simulink model "PSO_PDD_OLD"  (R2015a)
settings: Solver=ode4  StartTime=0.0  StopTime=16  FixedStep=0.1  RelTol=1e-3
model workspace: external: MAT-File co-effs.mat (data not in the file)
libraries: aerolibutil x7, vrlib x5, simulink x1, simulink_extras x1
settings Model: Creator=Nick  LastModifiedBy=Nick
settings DataIOCC: ReturnWorkspaceOutputs=on

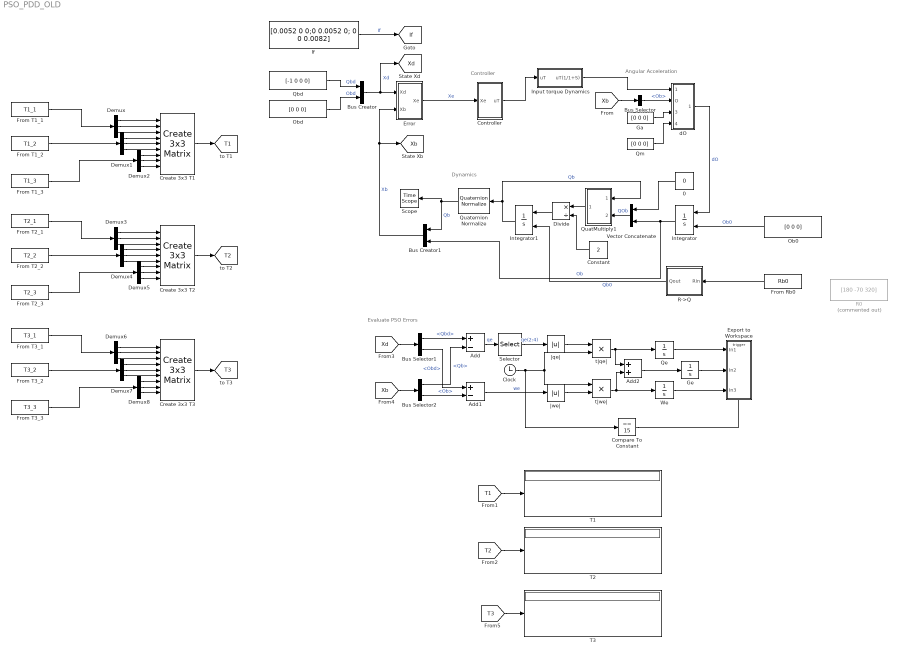
== system PSO_PDD_OLD ==
  note: Evaluate PSO Errors
  note: Dynamics
  note: Controller
  note: Angular Acceleration
  0 : Constant  Value=0
  Add : Sum  Inputs=+-
  Add1 : Sum  Inputs=+-
  Add2 : Sum
  Bus Creator : BusCreator  Inputs='Qbd','Obd'
  Bus Creator1 : BusCreator  Inputs='Qb','Ob'
  Bus Selector : BusSelector  OutputSignals=Ob
  Bus Selector1 : BusSelector  OutputSignals=Qbd,Obd
  Bus Selector2 : BusSelector  OutputSignals=Qb,Ob
  Clock : Clock
  Compare To Constant : simulink/Logic and Bit Operations/Compare To Constant  relop===  const=15  OutDataTypeStr=boolean
  Constant : Constant  Value=2
  Controller : Subsystem
  Create 3x3 T1 : aerolibutil/Create 3x3 Matrix
  Create 3x3 T2 : aerolibutil/Create 3x3 Matrix
  Create 3x3 T3 : aerolibutil/Create 3x3 Matrix
  Demux{,1..8} (9 alike) : Demux  Outputs=3
  Divide : Product  Inputs=*/
  Error : Subsystem
  Export to Workspace : Subsystem
  From Rb0 : FromWorkspace  VariableName=Rb0  SampleTime=0
  From T1_1 : FromWorkspace  VariableName=T1_1  SampleTime=0
  From T1_2 : FromWorkspace  VariableName=T1_2  SampleTime=0
  From T1_3 : FromWorkspace  VariableName=T1_3  SampleTime=0
  From T2_1 : FromWorkspace  VariableName=T2_1  SampleTime=0
  From T2_2 : FromWorkspace  VariableName=T2_2  SampleTime=0
  From T2_3 : FromWorkspace  VariableName=T2_3  SampleTime=0
  From T3_1 : FromWorkspace  VariableName=T3_1  SampleTime=0
  From T3_2 : FromWorkspace  VariableName=T3_2  SampleTime=0
  From T3_3 : FromWorkspace  VariableName=T3_3  SampleTime=0
  Ga : Constant  Value=[0 0 0]
  Ge : Integrator
  If : Constant  Value=[0.0052 0 0;0 0.0052 0; 0 0 0.0082]  VectorParams1D=off
  Input torque Dynamics : Subsystem
  Integrator : Integrator  InitialConditionSource=external
  Integrator1 : Integrator  InitialConditionSource=external
  Ob0 : Constant  Value=[0 0 0]
  Obd : Constant  Value=[0 0 0]
  Qbd : Constant  Value=[-1 0 0 0]
  Qe : Integrator
  Qm : Constant  Value=[0 0 0]
  QuatMultiply1 : Subsystem
  Quaternion Normalize : aerolibutil/Quaternion Normalize
  R->Q : Subsystem
  R0 : Constant  Commented=on  Value=[180 -70 320]
  Scope : TimeScope
  Selector : Selector  InputPortWidth=4  Indices=[2 3 4]
  T1 : Display
  T2 : Display
  T3 : Display
  Vector Concatenate : Concatenate
  We : Integrator
  dO : Subsystem
  t|qe| : Product
  t|we| : Product
  |qe| : Abs
  |we| : Abs
  tag scope: If=global, T1=global, T2=global, T3=global, Xb=global, Xd=global
  wires:
  Qbd/1 -> Bus Creator/1  "Qbd"
  Obd/1 -> Bus Creator/2  "Obd"
  Bus Creator/1 -> [Xd], Error/1(Xd)  "Xd"
  If/1 -> [If]  "If"
  Error/1(Xe) -> Controller/1(Xe)  "Xe"
  Controller/1(uT) -> Input torque Dynamics/1(uT)
  Input torque Dynamics/1(uT(1/1+S)) -> dO/1(uT)
  [Xb] -> Bus Selector/1
  Bus Selector/1 -> dO/2(O)  "<Ob>"
  Ga/1 -> dO/3(Ga)
  Qm/1 -> dO/4(Qm)
  dO/1(dO) -> Integrator/1  "dO"
  Integrator/1 -> Vector Concatenate/2, Bus Creator1/2  "Ob"
  Constant/1 -> Divide/2
  R->Q/1(Qout) -> Integrator1/2  "Qb0"
  Integrator1/1 -> Quaternion Normalize/1, QuatMultiply1/1(Q1 in)  "Qb"
  0/1 -> Vector Concatenate/1
  Vector Concatenate/1 -> QuatMultiply1/2(Q2 in)  "QOb"
  Divide/1 -> Integrator1/1
  QuatMultiply1/1(Qout) -> Divide/1
  Quaternion Normalize/1 -> Bus Creator1/1, Scope/1  "Qb"
  Bus Creator1/1 -> Error/2(Xb), [Xb]  "Xb"
  [Xb] -> Bus Selector2/1
  [Xd] -> Bus Selector1/1
  Bus Selector1/1 -> Add/1  "<Qbd>"
  Bus Selector1/2 -> Add1/1  "<Obd>"
  Bus Selector2/1 -> Add/2  "<Qb>"
  Bus Selector2/2 -> Add1/2  "<Ob>"
  Add/1 -> Selector/1  "qe"
  Clock/1 -> Compare To Constant/1, t|we|/1, t|qe|/2
  t|qe|/1 -> Qe/1, Add2/1
  Selector/1 -> |qe|/1  "qe(2:4)"
  |qe|/1 -> t|qe|/1
  |we|/1 -> t|we|/2
  t|we|/1 -> Add2/2, We/1
  Add1/1 -> |we|/1  "we"
  Add2/1 -> Ge/1
  Qe/1 -> Export to Workspace/1(In1)
  Ge/1 -> Export to Workspace/2(In2)
  We/1 -> Export to Workspace/3(In3)
  Compare To Constant/1 -> Export to Workspace/Trigger
  Ob0/1 -> Integrator/2  "Ob0"
  From Rb0/1 -> R->Q/1(Rin)
  From T1_2/1 -> Demux1/1
  From T1_1/1 -> Demux/1
  From T1_3/1 -> Demux2/1
  Demux/1 -> Create 3x3 T1/1
  Demux/2 -> Create 3x3 T1/2
  Demux/3 -> Create 3x3 T1/3
  Demux1/1 -> Create 3x3 T1/4
  Demux1/2 -> Create 3x3 T1/5
  Demux1/3 -> Create 3x3 T1/6
  Demux2/1 -> Create 3x3 T1/7
  Demux2/2 -> Create 3x3 T1/8
  Demux2/3 -> Create 3x3 T1/9
  Create 3x3 T1/1 -> [T1]
  From T2_2/1 -> Demux4/1
  From T2_1/1 -> Demux3/1
  From T2_3/1 -> Demux5/1
  Demux3/1 -> Create 3x3 T2/1
  Demux3/2 -> Create 3x3 T2/2
  Demux3/3 -> Create 3x3 T2/3
  Demux4/1 -> Create 3x3 T2/4
  Demux4/2 -> Create 3x3 T2/5
  Demux4/3 -> Create 3x3 T2/6
  Demux5/1 -> Create 3x3 T2/7
  Demux5/2 -> Create 3x3 T2/8
  Demux5/3 -> Create 3x3 T2/9
  Create 3x3 T2/1 -> [T2]
  From T3_2/1 -> Demux7/1
  From T3_1/1 -> Demux6/1
  From T3_3/1 -> Demux8/1
  Demux6/1 -> Create 3x3 T3/1
  Demux6/2 -> Create 3x3 T3/2
  Demux6/3 -> Create 3x3 T3/3
  Demux7/1 -> Create 3x3 T3/4
  Demux7/2 -> Create 3x3 T3/5
  Demux7/3 -> Create 3x3 T3/6
  Demux8/1 -> Create 3x3 T3/7
  Demux8/2 -> Create 3x3 T3/8
  Demux8/3 -> Create 3x3 T3/9
  Create 3x3 T3/1 -> [T3]
  [T1] -> T1/1
  [T2] -> T2/1
  [T3] -> T3/1

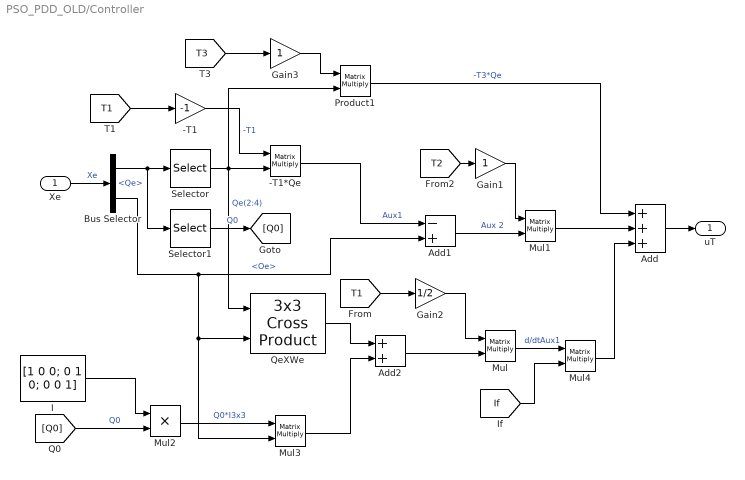
== system PSO_PDD_OLD/Controller ==
  Xe : Inport  PortDimensions=7
  -T1 : Gain  Gain=-1
  -T1*Qe : Product  Multiplication=Matrix(*)
  Add : Sum  Inputs=+++
  Add1 : Sum  Inputs=-+
  Add2 : Sum
  Bus Selector : BusSelector  OutputSignals=Qe,Oe
  Gain1 : Gain
  Gain2 : Gain  Gain=1/2
  Gain3 : Gain
  I : Constant  Value=[1 0 0; 0 1 0; 0 0 1]
  Mul{,1,3..4} (4 alike) : Product  Inputs=**  Multiplication=Matrix(*)
  Mul2 : Product  Inputs=**
  Product1 : Product  Multiplication=Matrix(*)
  QeXWe : aerolibutil/3x3 Cross Product
  Selector : Selector  InputPortWidth=4  Indices=[2 3 4]
  Selector1 : Selector  InputPortWidth=4  Indices=[1]
  uT : Outport  PortDimensions=3
  wires:
  Xe/1 -> Bus Selector/1  "Xe"
  Bus Selector/1 -> Selector1/1, Selector/1  "<Qe>"
  Selector/1 -> Product1/2, -T1*Qe/2, QeXWe/1  "Qe(2:4)"
  [T1] -> -T1/1
  -T1/1 -> -T1*Qe/1  "-T1"
  -T1*Qe/1 -> Add1/1  "Aux1"
  [T2] -> Gain1/1
  Add1/1 -> Mul1/2  "Aux 2"
  Gain1/1 -> Mul1/1
  Mul1/1 -> Add/2
  Bus Selector/2 -> Mul3/2, QeXWe/2, Add1/2  "<Oe>"
  Selector1/1 -> [Q0]  "Q0"
  I/1 -> Mul2/1
  [Q0] -> Mul2/2  "Q0"
  Mul2/1 -> Mul3/1  "Q0*I3x3"
  QeXWe/1 -> Add2/1
  Mul3/1 -> Add2/2
  Add2/1 -> Mul/2
  [T1] -> Gain2/1
  Gain2/1 -> Mul/1
  [T3] -> Gain3/1
  Gain3/1 -> Product1/1
  Product1/1 -> Add/1  "-T3*Qe"
  [If] -> Mul4/2
  Add/1 -> uT/1
  Mul/1 -> Mul4/1  "d/dtAux1"
  Mul4/1 -> Add/3

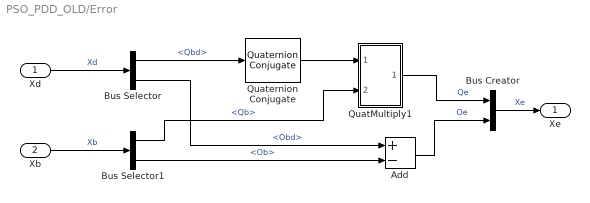
== system PSO_PDD_OLD/Error ==
  Xd : Inport
  Xb : Inport  Port=2  PortDimensions=7
  Add : Sum  Inputs=+-
  Bus Selector : BusSelector  OutputSignals=Qbd,Obd
  Bus Selector1 : BusSelector  OutputSignals=Qb,Ob
  Bus Creator : BusCreator  Inputs=2
  QuatMultiply1 : Subsystem
  Quaternion Conjugate : aerolibutil/Quaternion Conjugate
  Xe : Outport
  wires:
  Xd/1 -> Bus Selector/1  "Xd"
  Xb/1 -> Bus Selector1/1  "Xb"
  Bus Selector/1 -> Quaternion Conjugate/1  "<Qbd>"
  Bus Selector/2 -> Add/1  "<Obd>"
  QuatMultiply1/1(Qout) -> Bus Creator/1  "Qe"
  Add/1 -> Bus Creator/2  "Oe"
  Bus Creator/1 -> Xe/1  "Xe"
  Bus Selector1/1 -> QuatMultiply1/2(Q2 in)  "<Qb>"
  Quaternion Conjugate/1 -> QuatMultiply1/1(Q1 in)
  Bus Selector1/2 -> Add/2  "<Ob>"

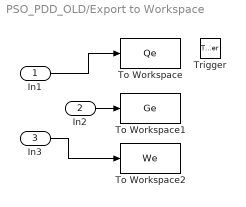
== system PSO_PDD_OLD/Export to Workspace ==
  In1 : Inport
  In2 : Inport  Port=2
  In3 : Inport  Port=3
  Trigger : TriggerPort  PortDimensions=1
  To Workspace : ToWorkspace  VariableName=Qe  SampleTime=-1
  To Workspace1 : ToWorkspace  VariableName=Ge  SampleTime=-1
  To Workspace2 : ToWorkspace  VariableName=We  SampleTime=-1
  wires:
  In1/1 -> To Workspace/1
  In2/1 -> To Workspace1/1
  In3/1 -> To Workspace2/1

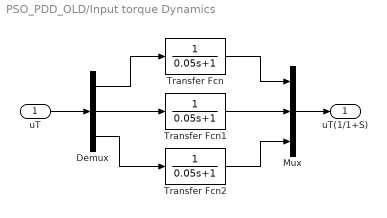
== system PSO_PDD_OLD/Input torque Dynamics ==
  uT : Inport  PortDimensions=3
  Demux : Demux  Outputs=3
  Mux : Mux  Inputs=3
  Transfer Fcn : TransferFcn  Denominator=[0.05 1]
  Transfer Fcn1 : TransferFcn  Denominator=[0.05 1]
  Transfer Fcn2 : TransferFcn  Denominator=[0.05 1]
  uT(1/1+S) : Outport  PortDimensions=3
  wires:
  uT/1 -> Demux/1
  Demux/1 -> Transfer Fcn/1
  Demux/2 -> Transfer Fcn1/1
  Demux/3 -> Transfer Fcn2/1
  Transfer Fcn/1 -> Mux/1
  Transfer Fcn1/1 -> Mux/2
  Transfer Fcn2/1 -> Mux/3
  Mux/1 -> uT(1/1+S)/1

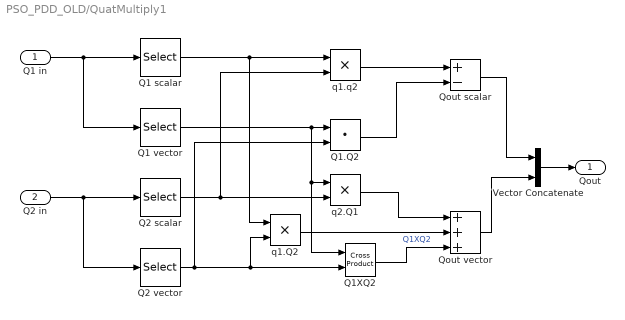
== system PSO_PDD_OLD/QuatMultiply1 ==
  Q1 in : Inport  PortDimensions=[4]
  Q2 in : Inport  Port=2  PortDimensions=[4]
  Q1 scalar : Selector  InputPortWidth=4  Indices=[1]
  Q1 vector : Selector  InputPortWidth=4  Indices=[2 3 4]
  Q1.Q2 : DotProduct  InputSameDT=on  OutDataTypeStr=Inherit: Inherit via internal rule
  Q1XQ2 : vrlib/Utilities/Cross Product
  Q2 scalar : Selector  InputPortWidth=4  Indices=[1]
  Q2 vector : Selector  InputPortWidth=4  Indices=[2 3 4]
  Qout scalar : Sum  Inputs=+-
  Qout vector : Sum  Inputs=+++
  Vector Concatenate : Concatenate
  q1.Q2 : Product
  q1.q2 : Product
  q2.Q1 : Product
  Qout : Outport  PortDimensions=[4]
  wires:
  Q1 in/1 -> Q1 vector/1, Q1 scalar/1
  Q2 in/1 -> Q2 vector/1, Q2 scalar/1
  Q1 scalar/1 -> q1.q2/1, q1.Q2/1
  Q2 scalar/1 -> q1.q2/2, q2.Q1/2
  Q1 vector/1 -> Q1.Q2/1, Q1XQ2/1, q2.Q1/1
  Q2 vector/1 -> Q1.Q2/2, Q1XQ2/2, q1.Q2/2
  q1.q2/1 -> Qout scalar/1
  Q1.Q2/1 -> Qout scalar/2
  q2.Q1/1 -> Qout vector/1
  q1.Q2/1 -> Qout vector/2
  Qout scalar/1 -> Vector Concatenate/1
  Qout vector/1 -> Vector Concatenate/2
  Vector Concatenate/1 -> Qout/1
  Q1XQ2/1 -> Qout vector/3  "Q1XQ2"

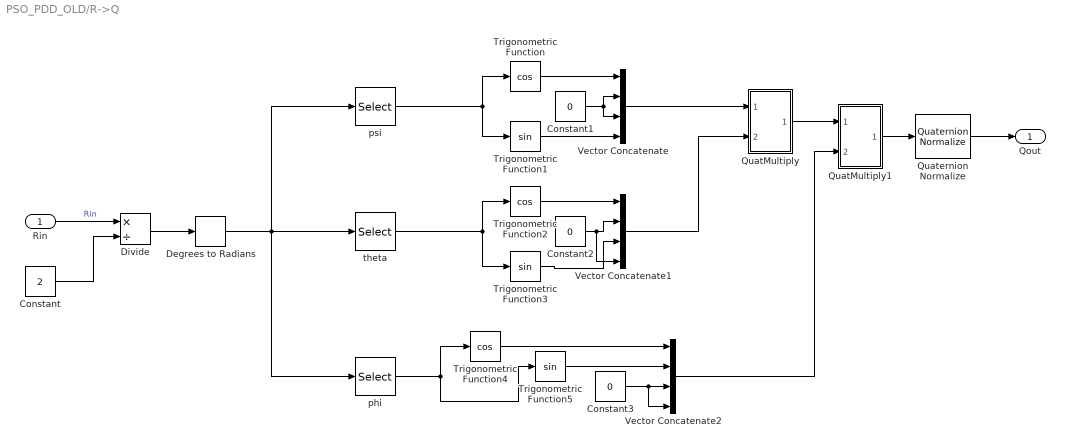
== system PSO_PDD_OLD/R->Q ==
  Rin : Inport  PortDimensions=3
  Constant : Constant  Value=2
  Constant1 : Constant  Value=0
  Constant2 : Constant  Value=0
  Constant3 : Constant  Value=0
  Degrees to Radians : simulink_extras/Transformations/Degrees to Radians
  Divide : Product  Inputs=*/
  QuatMultiply : Subsystem
  QuatMultiply1 : Subsystem
  Quaternion Normalize : aerolibutil/Quaternion Normalize
  Trigonometric Function : Trigonometry  Operator=cos
  Trigonometric Function1 : Trigonometry
  Trigonometric Function2 : Trigonometry  Operator=cos
  Trigonometric Function3 : Trigonometry
  Trigonometric Function4 : Trigonometry  Operator=cos
  Trigonometric Function5 : Trigonometry
  Vector Concatenate : Concatenate  NumInputs=4
  Vector Concatenate1 : Concatenate  NumInputs=4
  Vector Concatenate2 : Concatenate  NumInputs=4
  phi : Selector  InputPortWidth=3  Indices=[1]
  psi : Selector  InputPortWidth=3  Indices=[3]
  theta : Selector  InputPortWidth=3  Indices=[2]
  Qout : Outport  PortDimensions=[4]
  wires:
  Trigonometric Function/1 -> Vector Concatenate/1
  psi/1 -> Trigonometric Function1/1, Trigonometric Function/1
  Trigonometric Function1/1 -> Vector Concatenate/4
  Constant1/1 -> Vector Concatenate/3, Vector Concatenate/2
  Constant/1 -> Divide/2
  Rin/1 -> Divide/1  "Rin"
  Trigonometric Function2/1 -> Vector Concatenate1/1
  theta/1 -> Trigonometric Function3/1, Trigonometric Function2/1
  Constant2/1 -> Vector Concatenate1/4, Vector Concatenate1/2
  Trigonometric Function3/1 -> Vector Concatenate1/3
  Trigonometric Function4/1 -> Vector Concatenate2/1
  phi/1 -> Trigonometric Function5/1, Trigonometric Function4/1
  Trigonometric Function5/1 -> Vector Concatenate2/2
  Constant3/1 -> Vector Concatenate2/4, Vector Concatenate2/3
  Vector Concatenate/1 -> QuatMultiply/1(Q1 in)
  Vector Concatenate1/1 -> QuatMultiply/2(Q2 in)
  QuatMultiply/1(Qout) -> QuatMultiply1/1(Q1 in)
  Vector Concatenate2/1 -> QuatMultiply1/2(Q2 in)
  Divide/1 -> Degrees to Radians/1
  Degrees to Radians/1 -> phi/1, psi/1, theta/1
  QuatMultiply1/1(Qout) -> Quaternion Normalize/1
  Quaternion Normalize/1 -> Qout/1

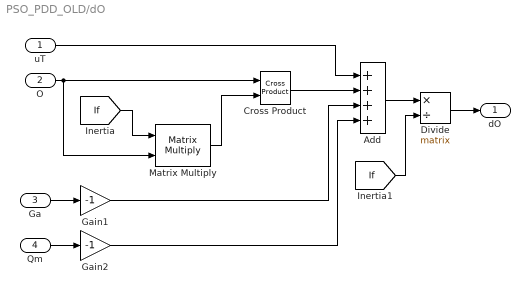
== system PSO_PDD_OLD/dO ==
  uT : Inport  PortDimensions=3
  O : Inport  Port=2  PortDimensions=3
  Ga : Inport  Port=3  PortDimensions=3
  Qm : Inport  Port=4  PortDimensions=3
  Add : Sum  Inputs=++++
  Cross Product : vrlib/Utilities/Cross Product
  Divide : Product  Inputs=*/  Multiplication=Matrix(*)
  Gain1 : Gain  Gain=-1
  Gain2 : Gain  Gain=-1
  Matrix Multiply : Product  Multiplication=Matrix(*)
  dO : Outport  PortDimensions=3
  wires:
  Divide/1 -> dO/1
  [If] -> Divide/2
  Ga/1 -> Gain1/1
  Qm/1 -> Gain2/1
  uT/1 -> Add/1
  Gain1/1 -> Add/3
  Gain2/1 -> Add/4
  Add/1 -> Divide/1
  [If] -> Matrix Multiply/1
  O/1 -> Cross Product/1, Matrix Multiply/2
  Matrix Multiply/1 -> Cross Product/2
  Cross Product/1 -> Add/2

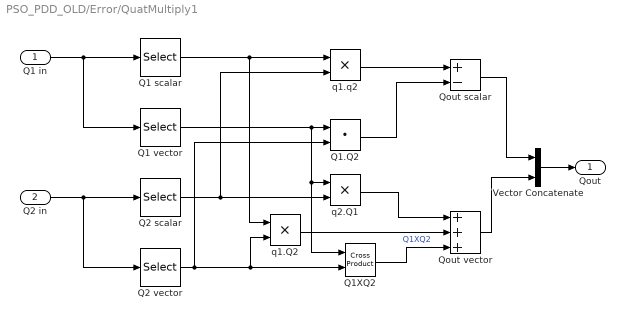
== system PSO_PDD_OLD/Error/QuatMultiply1 ==
  Q1 in : Inport  PortDimensions=[4]
  Q2 in : Inport  Port=2  PortDimensions=[4]
  Q1 scalar : Selector  InputPortWidth=4  Indices=[1]
  Q1 vector : Selector  InputPortWidth=4  Indices=[2 3 4]
  Q1.Q2 : DotProduct  InputSameDT=on  OutDataTypeStr=Inherit: Inherit via internal rule
  Q1XQ2 : vrlib/Utilities/Cross Product
  Q2 scalar : Selector  InputPortWidth=4  Indices=[1]
  Q2 vector : Selector  InputPortWidth=4  Indices=[2 3 4]
  Qout scalar : Sum  Inputs=+-
  Qout vector : Sum  Inputs=+++
  Vector Concatenate : Concatenate
  q1.Q2 : Product
  q1.q2 : Product
  q2.Q1 : Product
  Qout : Outport  PortDimensions=[4]
  wires:
  Q1 in/1 -> Q1 vector/1, Q1 scalar/1
  Q2 in/1 -> Q2 vector/1, Q2 scalar/1
  Q1 scalar/1 -> q1.q2/1, q1.Q2/1
  Q2 scalar/1 -> q1.q2/2, q2.Q1/2
  Q1 vector/1 -> Q1.Q2/1, Q1XQ2/1, q2.Q1/1
  Q2 vector/1 -> Q1.Q2/2, Q1XQ2/2, q1.Q2/2
  q1.q2/1 -> Qout scalar/1
  Q1.Q2/1 -> Qout scalar/2
  q2.Q1/1 -> Qout vector/1
  q1.Q2/1 -> Qout vector/2
  Qout scalar/1 -> Vector Concatenate/1
  Qout vector/1 -> Vector Concatenate/2
  Vector Concatenate/1 -> Qout/1
  Q1XQ2/1 -> Qout vector/3  "Q1XQ2"

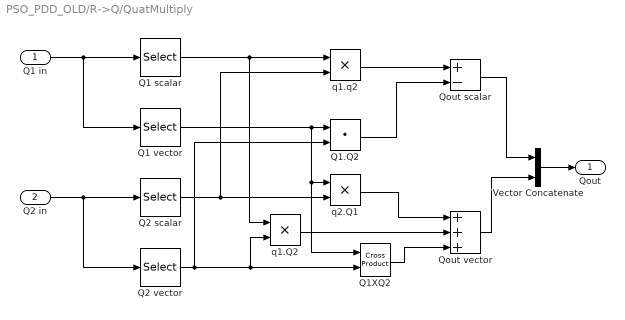
== system PSO_PDD_OLD/R->Q/QuatMultiply ==
  Q1 in : Inport  PortDimensions=[4]
  Q2 in : Inport  Port=2  PortDimensions=[4]
  Q1 scalar : Selector  InputPortWidth=4  Indices=[1]
  Q1 vector : Selector  InputPortWidth=4  Indices=[2 3 4]
  Q1.Q2 : DotProduct  InputSameDT=on  OutDataTypeStr=Inherit: Inherit via internal rule
  Q1XQ2 : vrlib/Utilities/Cross Product
  Q2 scalar : Selector  InputPortWidth=4  Indices=[1]
  Q2 vector : Selector  InputPortWidth=4  Indices=[2 3 4]
  Qout scalar : Sum  Inputs=+-
  Qout vector : Sum  Inputs=+++
  Vector Concatenate : Concatenate
  q1.Q2 : Product
  q1.q2 : Product
  q2.Q1 : Product
  Qout : Outport  PortDimensions=[4]
  wires:
  Q1 in/1 -> Q1 vector/1, Q1 scalar/1
  Q2 in/1 -> Q2 vector/1, Q2 scalar/1
  Q1 scalar/1 -> q1.q2/1, q1.Q2/1
  Q2 scalar/1 -> q1.q2/2, q2.Q1/2
  Q1 vector/1 -> Q1.Q2/1, q2.Q1/1, Q1XQ2/1
  Q2 vector/1 -> Q1.Q2/2, q1.Q2/2, Q1XQ2/2
  q1.q2/1 -> Qout scalar/1
  Q1.Q2/1 -> Qout scalar/2
  q2.Q1/1 -> Qout vector/1
  q1.Q2/1 -> Qout vector/2
  Q1XQ2/1 -> Qout vector/3
  Qout scalar/1 -> Vector Concatenate/1
  Qout vector/1 -> Vector Concatenate/2
  Vector Concatenate/1 -> Qout/1

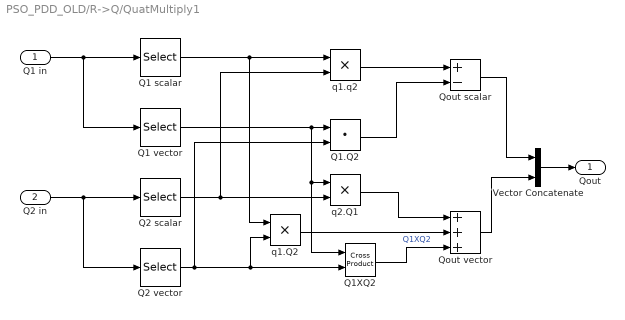
== system PSO_PDD_OLD/R->Q/QuatMultiply1 ==
  Q1 in : Inport  PortDimensions=[4]
  Q2 in : Inport  Port=2  PortDimensions=[4]
  Q1 scalar : Selector  InputPortWidth=4  Indices=[1]
  Q1 vector : Selector  InputPortWidth=4  Indices=[2 3 4]
  Q1.Q2 : DotProduct  InputSameDT=on  OutDataTypeStr=Inherit: Inherit via internal rule
  Q1XQ2 : vrlib/Utilities/Cross Product
  Q2 scalar : Selector  InputPortWidth=4  Indices=[1]
  Q2 vector : Selector  InputPortWidth=4  Indices=[2 3 4]
  Qout scalar : Sum  Inputs=+-
  Qout vector : Sum  Inputs=+++
  Vector Concatenate : Concatenate
  q1.Q2 : Product
  q1.q2 : Product
  q2.Q1 : Product
  Qout : Outport  PortDimensions=[4]
  wires:
  Q1 in/1 -> Q1 vector/1, Q1 scalar/1
  Q2 in/1 -> Q2 vector/1, Q2 scalar/1
  Q1 scalar/1 -> q1.q2/1, q1.Q2/1
  Q2 scalar/1 -> q1.q2/2, q2.Q1/2
  Q1 vector/1 -> Q1.Q2/1, Q1XQ2/1, q2.Q1/1
  Q2 vector/1 -> Q1.Q2/2, Q1XQ2/2, q1.Q2/2
  q1.q2/1 -> Qout scalar/1
  Q1.Q2/1 -> Qout scalar/2
  q2.Q1/1 -> Qout vector/1
  q1.Q2/1 -> Qout vector/2
  Qout scalar/1 -> Vector Concatenate/1
  Qout vector/1 -> Vector Concatenate/2
  Vector Concatenate/1 -> Qout/1
  Q1XQ2/1 -> Qout vector/3  "Q1XQ2"
